simulink model "p2b2"  (R2023b)
settings: Solver=VariableStepAuto  StartTime=0.0  StopTime=15  RelTol=1e-3
libraries: simulink_extras x3
settings Model: Creator=tanvi  LastModifiedBy=tanvi

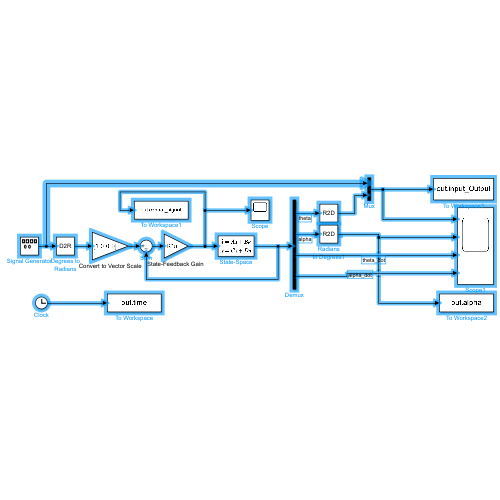
[thumbnail: Simulink's stored preview of the top-level diagram]
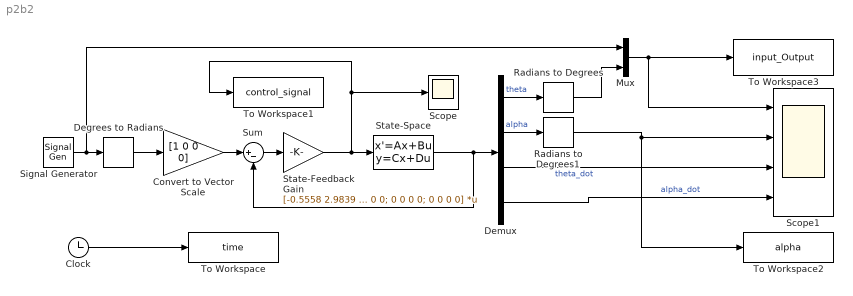
== system p2b2 ==
  Clock : Clock
  Convert to Vector Scale : Gain  Gain=[1 0 0 0]
  Degrees to Radians : simulink_extras/Transformations/Degrees to Radians
  Demux : Demux
  Mux : Mux  Inputs=2
  Radians to Degrees : simulink_extras/Transformations/Radians to Degrees
  Radians to Degrees1 : simulink_extras/Transformations/Radians to Degrees
  Scope : Scope
  Scope1 : Scope  NumInputPorts=4
  Signal Generator : SignalGenerator  WaveForm=square  Amplitude=20  Frequency=0.1
  "State-Feedback Gain " : Gain  Gain=[-0.5558 2.9839 -0.3545 0.2418; 0 0 0 0; 0 0 0 0; 0 0 0 0]  Multiplication=Matrix(K*u)
  State-Space : StateSpace  A=[0 0 1 0; 0 0 0 1; 261 -1328.8 113.1 -115.4; 422.8 -2078.9 183.3 -188.7]  B=[0 0 0 0; 0 0 0 0; 469.5697 0 0 0; 760.6579 0 0 0]  C=[1 0 0 0; 0 1 0 0; 0 0 0 0; 0 0 0 0]  D=[0 0 0 0; 0 0 0 0; 0 0 0 0; 0 0 0 0]  InitialCondition=0
  Sum : Sum  Inputs=|+-
  To Workspace : ToWorkspace  VariableName=time  SampleTime=-1
  To Workspace1 : ToWorkspace  VariableName=control_signal  SampleTime=-1
  To Workspace2 : ToWorkspace  VariableName=alpha  SampleTime=-1
  To Workspace3 : ToWorkspace  VariableName=input_Output  SampleTime=-1
  wires:
  State-Space/1 -> Sum/2, Demux/1
  Degrees to Radians/1 -> Convert to Vector Scale/1
  Convert to Vector Scale/1 -> Sum/1
  Demux/4 -> Scope1/4  "alpha_dot"
  Demux/2 -> Radians to Degrees1/1  "alpha"
  Demux/1 -> Radians to Degrees/1  "theta"
  Sum/1 -> "State-Feedback Gain "/1
  Clock/1 -> To Workspace/1
  Mux/1 -> Scope1/1, To Workspace3/1
  Radians to Degrees1/1 -> To Workspace2/1, Scope1/2
  "State-Feedback Gain "/1 -> To Workspace1/1, Scope/1, State-Space/1
  Signal Generator/1 -> Mux/1, Degrees to Radians/1
  Radians to Degrees/1 -> Mux/2
  Demux/3 -> Scope1/3  "theta_dot"
